simulink model "DFIG_wind_turbine_model"  (R2013a)
settings: Solver=ode45  StartTime=0.0  StopTime=10.0  RelTol=1e-3
undefined symbols (not defined in the file): c1, c2, c3, c4, c5, c6
libraries: powerlib x36
settings Model: Creator=Görkem  LastModifiedBy=Görkem

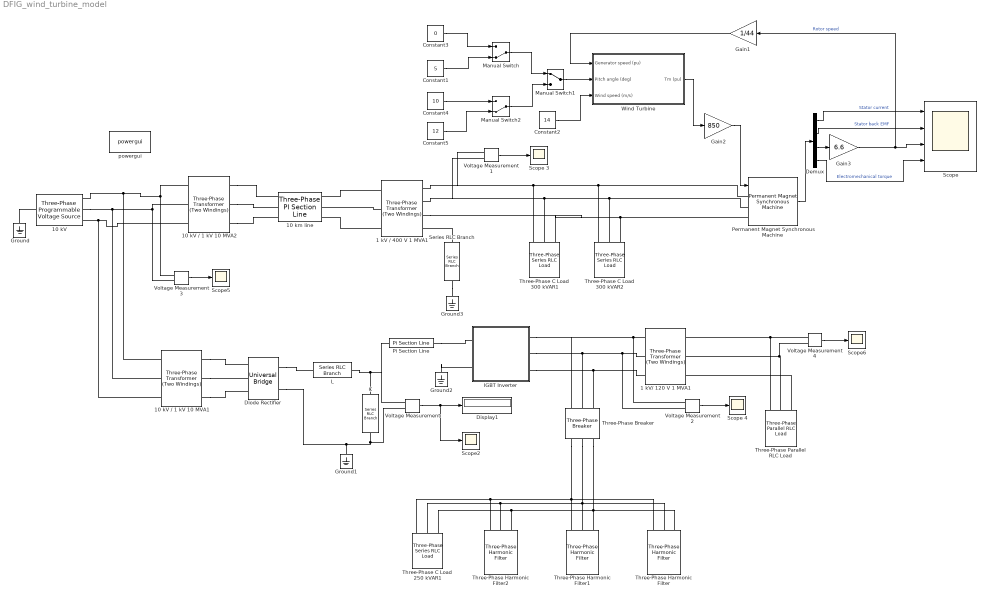
== system DFIG_wind_turbine_model ==
  1 kV / 400 V 1 MVA1 : powerlib/Elements/Three-Phase Transformer (Two Windings)  Winding1Connection=Y  UNITS=SI  NominalPower=[ 1000e3, 50 ]  Winding1=[1000 0.0023104 0.00029417]  Winding2Connection=Yn  Winding2=[400 0.0017328 0.00022063]  SetSaturation=off  Rm=577.6  Lm=1.8386  Saturation=[0 0;1.2892 2.3703;537.17 3.0024]  Hysteresis=off  DataFile='hysteresis'  SetInitialFlux=off  InitialFluxes=[1.5802 -1.5802 1.3827]  Measurements=None  MoreParameters=off  BreakLoop=off  DataType=on  TransfoNumber=1
  1 kV/ 120 V 1 MVA1 : powerlib/Elements/Three-Phase Transformer (Two Windings)  Winding1Connection=Yg  UNITS=SI  NominalPower=[ 1000000, 50 ]  Winding1=[1000 0.08712 0.011092]  Winding2Connection=Y  Winding2=[120 0.0008664 0.00011031]  SetSaturation=off  Rm=21780  Lm=69.328  Saturation=[0 0;0.29691 20.584;123.71 26.073]  Hysteresis=off  DataFile='hysteresis'  SetInitialFlux=off  InitialFluxes=[13.723 -13.723 12.007]  Measurements=None  MoreParameters=off  BreakLoop=off  DataType=on  TransfoNumber=1
  10 kV : powerlib/Electrical Sources/Three-Phase Programmable Voltage Source  PositiveSequence="[10000  0 50]"  VariationEntity=None  VariationType=Table of time-amplitude pairs  VariationTypeAlt=Step  VariationStep=0.5  VariationRate=10  VariationMagnitude=0.3  VariationFrequency=2  VariationTiming=[1 2]  VariationPhaseA=off  Amplitudes=[1 0.8 1.2 1.0]  TimeValues=[0 0.1 0.15 0.2]  HarmonicGeneration=off  HarmonicA=[3 0.2 -25 0]  HarmonicB=[2 0.15 35 2]  Timing="[0.05  3]"  BusType=swing  Pref=0  Qref=0  Qmin=-inf  Qmax=inf
  10 kV / 1 kV 10 MVA1 : powerlib/Elements/Three-Phase Transformer (Two Windings)  Winding1Connection=Y  UNITS=SI  NominalPower=[ 10e6, 50 ]  Winding1=[10000 0.0023104 0.00029417]  Winding2Connection=Y  Winding2=[1000 0.0017328 0.00022063]  SetSaturation=off  Rm=577.6  Lm=1.8386  Saturation=[0 0;1.2892 2.3703;537.17 3.0024]  Hysteresis=off  DataFile='hysteresis'  SetInitialFlux=off  InitialFluxes=[1.5802 -1.5802 1.3827]  Measurements=None  MoreParameters=off  BreakLoop=off  DataType=on  TransfoNumber=1
  10 kV / 1 kV 10 MVA2 : powerlib/Elements/Three-Phase Transformer (Two Windings)  Winding1Connection=Y  UNITS=SI  NominalPower=[ 10e6, 50 ]  Winding1=[10000 0.0023104 0.00029417]  Winding2Connection=Y  Winding2=[1000 0.0017328 0.00022063]  SetSaturation=off  Rm=577.6  Lm=1.8386  Saturation=[0 0;1.2892 2.3703;537.17 3.0024]  Hysteresis=off  DataFile='hysteresis'  SetInitialFlux=off  InitialFluxes=[1.5802 -1.5802 1.3827]  Measurements=None  MoreParameters=off  BreakLoop=off  DataType=on  TransfoNumber=1
  "10 km line " : powerlib/Elements/Three-Phase PI Section Line  LConnTagsString=a|b|c  RConnTagsString=A|B|C  Frequency=50  Resistances=[ 0.01273 0.3864]  Inductances="[ 0.9337e-3  4.1264e-3]"  Capacitances=[12.74e-9 7.751e-9]  Length=100
  C : powerlib/Elements/Series RLC Branch  LConnTagsString=__new0  RConnTagsString=__new0  BranchType=C  Resistance=1  Inductance=1e-3  SetiL0=off  InitialCurrent=0  Capacitance=0.01  Setx0=off  InitialVoltage=0  Measurements=None
  Constant1 : Constant  Value=5
  Constant2 : Constant  Value=14
  Constant3 : Constant  Value=0
  Constant4 : Constant  Value=10
  Constant5 : Constant  Value=12
  Demux : Demux
  Diode Rectifier : powerlib/Power Electronics/Universal Bridge  Arms=3  SnubberResistance=1e5  SnubberCapacitance=inf  Device=Diodes  Ron=1e-3  Lon=0  ForwardVoltages="[  0  0  ]"  ForwardVoltage=0  GTOparameters=[ 10e-6 , 20e-6 ]  IGBTparameters=[ 1e-6 , 2e-6 ]  Measurements=None  Measurements_2=None  converterType=Rectifier
  Display1 : Display
  Gain1 : Gain  Gain=1/44
  Gain2 : Gain  Gain=850
  Gain3 : Gain  Gain=6.6
  Ground{,1..3} (4 alike) : powerlib/Elements/Ground  LConnTagsString=a
  IGBT Inverter : Subsystem
  L : powerlib/Elements/Series RLC Branch  LConnTagsString=__new0  RConnTagsString=__new0  BranchType=L  Resistance=1  Inductance=3.8e-3  SetiL0=off  InitialCurrent=0  Capacitance=1e-6  Setx0=off  InitialVoltage=0  Measurements=None
  Manual Switch : ManualSwitch  CurrentSetting=0
  Manual Switch1 : ManualSwitch
  Manual Switch2 : ManualSwitch  CurrentSetting=0
  Permanent Magnet Synchronous Machine : powerlib/Machines/Permanent Magnet Synchronous Machine  NbPhases=3  FluxDistribution=Sinusoidal  RotorType=Round  MechanicalLoad=Torque Tm  PresetModel=No  ShowDetailedParameters=on  Resistance=0.0918  Inductance=8.5e-3  dqInductances=[8.5e-3,8.5e-3]  La=0.000975  MachineConstant=Flux linkage established by magnets (V.s)  Flux=0.1688  VoltageCst=122.4677  TorqueCst=1.0128  Flat=120  Mechanical=[0.003945 0.0004924 4 0]  PolePairs=4  InitialConditions=[0,0, 0,0]  InitialConditions5ph=[0 0 0 0 0 0]  TsPowergui=0  TsBlock=-1  RefAngle=90 degrees behind phase A axis (modified Park)
  Pi Section Line : powerlib/Elements/Pi Section Line  LConnTagsString=__new0  RConnTagsString=__new0  Frequency=50  Resistance=0.01273  Inductance=0.9337e-3  Capacitance=12.74e-9  Length=10  PiSections=1  Measurements=None
      settings: AttributesFormatString=\n
  Scope : Scope  NumInputPorts=4
      settings: YMin=-50000~-100000~-5~-5  YMax=50000~100000~5~5
  Scope 3 : Scope
      settings: SaveName=ScopeData3
  Scope 4 : Scope
      settings: SaveName=ScopeData4
  Scope2 : Scope
      settings: SaveName=ScopeData2
  Scope5 : Scope
      settings: SaveName=ScopeData5
  Scope6 : Scope
      settings: SaveName=ScopeData6
  Series RLC Branch : powerlib/Elements/Series RLC Branch  LConnTagsString=__new0  RConnTagsString=__new0  BranchType=R  Resistance=66  Inductance=1e-3  SetiL0=off  InitialCurrent=0  Capacitance=1e-6  Setx0=off  InitialVoltage=0  Measurements=None
  Three-Phase C Load 250 kVAR1 : powerlib/Elements/Three-Phase Series RLC Load  LConnTagsString=A|B|C  Configuration=Y (grounded)  NominalVoltage=1000  NominalFrequency=50  ActivePower=0  InductivePower=0  CapacitivePower=500000  Measurements=None  LoadType=constant Z
  Three-Phase C Load 300 kVAR1 : powerlib/Elements/Three-Phase Series RLC Load  LConnTagsString=A|B|C  Configuration=Y (floating)  NominalVoltage=380  NominalFrequency=50  ActivePower=0  InductivePower=0  CapacitivePower=300e3  Measurements=None  LoadType=constant Z
  Three-Phase C Load 300 kVAR2 : powerlib/Elements/Three-Phase Series RLC Load  LConnTagsString=A|B|C  Configuration=Y (floating)  NominalVoltage=380  NominalFrequency=50  ActivePower=0  InductivePower=0  CapacitivePower=300e3  Measurements=None  LoadType=constant Z
  Three-Phase Harmonic Filter : powerlib/Elements/Three-Phase Harmonic Filter  LConnTagsString=A|B|C  FilterType=Double-tuned  FilterConnection=Y (grounded)  ParNom=[1000 50]  Qc=500000  Fr=[5*60]  Frd=[11*50 13*50]  Q=16  Measurements=None
      settings: AttributesFormatString=\n
  Three-Phase Harmonic Filter1 : powerlib/Elements/Three-Phase Harmonic Filter  LConnTagsString=A|B|C  FilterType=C-type High-pass  FilterConnection=Y (grounded)  ParNom=[1000 50]  Qc=500000  Fr=[3*50]  Frd=[11*50 13*50]  Q=16  Measurements=None
      settings: AttributesFormatString=\n
  Three-Phase Harmonic Filter2 : powerlib/Elements/Three-Phase Harmonic Filter  LConnTagsString=A|B|C  FilterType=High-pass  FilterConnection=Y (grounded)  ParNom=[1000 50]  Qc=500000  Fr=[24*50]  Frd=[11*50 13*50]  Q=16  Measurements=None
      settings: AttributesFormatString=\n
  Three-Phase Parallel RLC Load : powerlib/Elements/Three-Phase Parallel RLC Load  LConnTagsString=A|B|C  Configuration=Y (grounded)  NominalVoltage=380  NominalFrequency=50  ActivePower=50e3  InductivePower=600  CapacitivePower=500  Measurements=None  LoadType=constant Z
  Three-Phase Breaker : powerlib/Elements/Three-Phase Breaker  InitialState=closed  SwitchA=on  SwitchB=on  SwitchC=on  SwitchTimes="[4/60  10/60]"  External=off  BreakerResistance=0.001  SnubberResistance=1e6  SnubberCapacitance=inf  Measurements=None
  Voltage Measurement{,1..4} (5 alike) : powerlib/Measurements/Voltage Measurement  PhasorSimulation=off  OutputType=Complex  PSBequivalent=0
  Wind Turbine : Subsystem  DialogController=POWERSYS.PowerSysDialog  mask(Wind Turbine){Pnom=50000, Pelec_base=56800, wind_base=14, P_wind_base=1, speed_nom=1, pitch_angle=0, DisplayTurbChar=off, c1_c6=[0.51763          116          0.4            5           21     0.006795], cp_nom=0.48, lambda_nom=8.1}
      mask prompts: Pnom "Nominal mechanical output power (W):"; Pelec_base "Base power of the electrical generator (VA):"; wind_base "Base wind speed (m/s):"; P_wind_base "Maximum power at base wind speed (pu of nominal mechanical power):"; speed_nom "Base rotational speed (p.u. of base generator speed):"; pitch_angle "Pitch angle beta to display wind-turbine power characteristics (beta >=0)  (deg):"; DisplayTurbChar "Display wind turbine power characteristics"
      mask help:
      | This block implements a variable pitch wind turbine model. The performance coefficient Cp of the turbine is the mechanical output power of the turbine divided by wind power and a function of wind speed, rotational speed, and pitch angle (beta). Cp reaches its maximum value at zero beta. Select the wind-turbine power characteristics display to plot the turbine characteristics at the specified pitch angle.
      |
      | The first input is the generator speed in per unit of the generator base speed. For a synchronous or asynchronous generator, the base speed is the synchronous speed. For a permanent-magnet generator, the base speed is defined as the speed producing nominal voltage at  no load. The second input is the blade pitch angle (beta) in degrees. The third input is the wind speed in m/s.
      |
      | The output is the torque applied to the generator shaft in per unit of the generator ratings.
      |
      | The turbine inertia must be added to the generator inertia.
      mask init:
      | %Wind turbine typical characteristic data
      | %c2=116;c3=0.4;c4=5;c5=21;
      | %Computation of c1 and c6 for lambda_nom et cpmax
      | %lambda_nom=8.1;
      | %cp_max=0.48;
      | %cp_nom=cp_max;
      | 
      | %lambda_i_nom=1/(1/lambda_nom-0.035);
      | %k_nom=-(c2*c5/lambda_i_nom-c4*c5-c2)*exp(-c5/lambda_i_nom)/lambda_nom^2;
      | %c1=cp_max/((c2/lambda_i_nom-c4)*exp(-c5/lambda_i_nom)+k_nom*lambda_nom);
      | %c6=k_nom*c1;
      | power_initmask();
      mask Help: helpview(psbhelp);
      mask Callback Pnom:
      | ParVisible={'on','on','on','on','on','on','on','off','off','off',};
      | set_param(gcb,'MaskVisibilities',ParVisible);
      | c1_c6=str2num(get_param(gcb,'c1_c6'));
      | c1=c1_c6(1);c2=c1_c6(2);c3=c1_c6(3);c4=c1_c6(4);c5=c1_c6(5);c6=c1_c6(6);
      mask Callback DisplayTurbChar:
      | DisplayTurbChar=get_param(gcb,'DisplayTurbChar');
      | 
      | if strcmp(DisplayTurbChar,'on')
      |     fig_num=figure;
      | 	clf(fig_num);
      | 	[speed_nom,wind_base,P_wind_base,pitch_angle]=getSPSmaskvalues(gcb,{'speed_nom','wind_base','P_wind_base','pitch_angle'});
      | 	[c1_c6,lambda_nom,cp_nom]=getSPSmaskvalues(gcb,{'c1_c6','lambda_nom','cp_nom'});
      | 	c1=c1_c6(1);c2=c1_c6(2);c3=c1_c6(3);c4=c1_c6(4);c5=c1_c6(5);c6=c1_c6(6);
      | 
      | 	%Wind turbine typical characteristic data
      |     %c2=116;c3=0.4;c4=5;c5=21;
      |     %Computation of c1 and c6 for lambda_nom et cpmax
      |     %lambda_nom=8.1;
      |     %cp_max=0.48;
      |     %cp_nom=cp_max;
      | 
      |     %lambda_i_nom=1/(1/lambda_nom-0.035);
      |     %k_nom=-(c2*c5/lambda_i_nom-c4*c5-c2)*exp(-c5/lambda_i_nom)/lambda_nom^2;
      |     %c1=cp_max/((c2/lambda_i_nom-c4)*exp(-c5/lambda_i_nom)+k_nom*lambda_nom);
      |     %c6=k_nom*c1;
      | 
      | 	wr_elec_pu=1e-3:0.01:1.5;;
      |     wr_mec_pu=wr_elec_pu/speed_nom;
      |     wind_max=ceil((1.2/P_wind_base)^(1/3)*wind_base);
      |     wind_min=round(((0.1)/P_wind_base)^(1/3)*wind_base);
      |     wind1=wind_min:(wind_base-wind_min)/5:wind_base;
      |     wind2=wind_base+(wind_base-wind_min)/5:(wind_base-wind_min)/5:wind_max;
      |     wind_pu=[wind1 wind2]/wind_base;
      | 
      |     for k=1:length(wind_pu)
      |         for i=1:length(wr_mec_pu);
      |             lambda_pu=wr_mec_pu(i)/wind_pu(k);
      |             lambda=lambda_pu*lambda_nom;
      |             lambda_i=1/(1/(lambda+0.08*pitch_angle)-0.035/(pitch_angle^3+1));
      |             cp=c1*(c2/lambda_i-c3*pitch_angle-c4)*exp(-c5/lambda_i)+c6*lambda;
      |             cp_pu=cp/cp_nom;
      |             Pwind_pu(k,i)=wind_pu(k)^3*cp_pu*P_wind_base;
      |         end
      |     end
      |     for k=1:length(wind_pu)
      |         plot(wr_elec_pu,Pwind_pu(k,:))
      |         hold on
      |     end
      | 
      |     plot([speed_nom,speed_nom,0],[0,P_wind_base,P_wind_base],'r--')
      |     text(speed_nom+0.01,0+0.05,sprintf('%0.4g pu',speed_nom))
      |     text(0.01,P_wind_base+0.05,sprintf('Max. power at base wind speed (%0.4g m/s) and beta = 0 deg',wind_base))
      |     for i=1:length(wind_pu),
      |         p_max(i)=max(Pwind_pu(i,:));
      |         speed(i)=wr_elec_pu(find(Pwind_pu(i,:)==p_max(i)));
      |         text(speed(i),p_max(i),sprintf('%0.4g m/s',wind_pu(i)*wind_base))
      |     end
      |     plot([0 max(wr_elec_pu)],[0 0],'--')
      | 
      |     xlabel('Turbine speed (pu of nominal generator speed)')
      |     ylabel('Turbine output power (pu of nominal mechanical power)')
      |     title(sprintf('Turbine Power Characteristics (Pitch angle beta = %0.4g deg)',pitch_angle))
      |     axis([0 max(wr_elec_pu) min(Pwind_pu(1,:)) max(P_wind_base+0.1,max(wind_pu)^3*P_wind_base+0.1)])
      |     set_param(gcb,'DisplayTurbChar','off')
      | end
      mask Display: disp('');
  powergui : powerlib/powergui  Priority=1  SimulationMode=Discrete  SolverType=Tustin  SampleTime=250e-6  frequency=60  SPID=off  DisableSnubberDevices=off  DisableRonSwitches=off  DisableVfSwitches=off  SwTol=0  Interpol=off  DisplayEquations=off  frequencyindice=50  Pbase=100e6  ErrMax=1e-4  Iterations=50  UnitsV=kV  UnitsW=MW  FunctionMessages=on  echomessages=off  HookPort=off  EnableUseOfTLC=off  x0status=blocks  RestoreLinks=warning  ResistiveCurrentMeasurement=off  Frange=[0:2:500]  Ylog=off  Xlog=on  ShowGrid=off  save=off  variable=ZData  ZoomFFT=off  StartTime=0.0  cycles=1  DisplayStyle=1  fundamental=60  FreqAxis=off  MaxFrequency=1000  frequencyindicesteady=1  RmsSteady=1  display=off  Ts=0  methode=off
  wires:
  Demux/3 -> Gain3/1
  Manual Switch1/1 -> Wind Turbine/2(Pitch angle (deg))
  Permanent Magnet Synchronous Machine/1 -> Demux/1
  Constant2/1 -> Wind Turbine/3(Wind speed (m/s))
  Wind Turbine/1(Tm (pu)) -> Gain2/1
  Gain1/1 -> Wind Turbine/1(Generator speed (pu))
  Demux/1 -> Scope/1  "Stator current"
  Demux/2 -> Scope/2  "Stator back EMF"
  Demux/4 -> Scope/4  "Electromechanical torque"
  Voltage Measurement/1 -> Display1/1, Scope2/1
  Gain2/1 -> Permanent Magnet Synchronous Machine/1
  Voltage Measurement2/1 -> Scope 4/1
  Voltage Measurement4/1 -> Scope6/1
  Voltage Measurement1/1 -> Scope 3/1
  Voltage Measurement3/1 -> Scope5/1
  Gain3/1 -> Scope/3, Gain1/1  "Rotor speed"
  Constant1/1 -> Manual Switch/2
  Constant3/1 -> Manual Switch/1
  Manual Switch/1 -> Manual Switch1/1
  Constant4/1 -> Manual Switch2/1
  Constant5/1 -> Manual Switch2/2
  Manual Switch2/1 -> Manual Switch1/2
  connections:
  L/RConn1 -- Pi Section Line/LConn1 -- Voltage Measurement/LConn1 -- C/LConn1
  Ground1/LConn1 -- Voltage Measurement/LConn2 -- C/RConn1 -- Diode Rectifier/RConn2
  Ground/LConn1 -- 10 kV/LConn1
  Pi Section Line/RConn1 -- IGBT Inverter/LConn1
  Ground2/LConn1 -- IGBT Inverter/LConn2
  Permanent Magnet Synchronous Machine/LConn2 -- Three-Phase C Load 300 kVAR2/LConn2 -- 1 kV / 400 V 1 MVA1/RConn2 -- Voltage Measurement1/LConn2 -- Three-Phase C Load 300 kVAR1/LConn2
  Three-Phase C Load 300 kVAR2/LConn3 -- Three-Phase C Load 300 kVAR1/LConn3 -- 1 kV / 400 V 1 MVA1/RConn3 -- Permanent Magnet Synchronous Machine/LConn3
  Three-Phase Parallel RLC Load/LConn2 -- Voltage Measurement4/LConn2 -- 1 kV/ 120 V 1 MVA1/RConn2
  Three-Phase Parallel RLC Load/LConn3 -- 1 kV/ 120 V 1 MVA1/RConn3
  Three-Phase Parallel RLC Load/LConn1 -- Voltage Measurement4/LConn1 -- 1 kV/ 120 V 1 MVA1/RConn1
  Voltage Measurement2/LConn1 -- IGBT Inverter/RConn1 -- Three-Phase Breaker/LConn1 -- 1 kV/ 120 V 1 MVA1/LConn1
  IGBT Inverter/RConn2 -- Three-Phase Breaker/LConn2 -- Voltage Measurement2/LConn2 -- 1 kV/ 120 V 1 MVA1/LConn2
  IGBT Inverter/RConn3 -- Three-Phase Breaker/LConn3 -- 1 kV/ 120 V 1 MVA1/LConn3
  Diode Rectifier/RConn1 -- L/LConn1
  Permanent Magnet Synchronous Machine/LConn1 -- Three-Phase C Load 300 kVAR2/LConn1 -- Voltage Measurement1/LConn1 -- 1 kV / 400 V 1 MVA1/RConn1 -- Three-Phase C Load 300 kVAR1/LConn1
  Three-Phase C Load 250 kVAR1/LConn1 -- Three-Phase Breaker/RConn1 -- Three-Phase Harmonic Filter1/LConn1 -- Three-Phase Harmonic Filter/LConn1 -- Three-Phase Harmonic Filter2/LConn1
  Three-Phase C Load 250 kVAR1/LConn2 -- Three-Phase Harmonic Filter2/LConn2 -- Three-Phase Breaker/RConn2 -- Three-Phase Harmonic Filter1/LConn2 -- Three-Phase Harmonic Filter/LConn2
  Three-Phase C Load 250 kVAR1/LConn3 -- Three-Phase Harmonic Filter2/LConn3 -- Three-Phase Breaker/RConn3 -- Three-Phase Harmonic Filter1/LConn3 -- Three-Phase Harmonic Filter/LConn3
  10 kV/RConn1 -- 10 kV / 1 kV 10 MVA1/LConn1 -- 10 kV / 1 kV 10 MVA2/LConn1 -- Voltage Measurement3/LConn1
  10 kV/RConn2 -- 10 kV / 1 kV 10 MVA1/LConn2 -- Voltage Measurement3/LConn2 -- 10 kV / 1 kV 10 MVA2/LConn2
  10 kV / 1 kV 10 MVA2/LConn3 -- 10 kV / 1 kV 10 MVA1/LConn3 -- 10 kV/RConn3
  1 kV / 400 V 1 MVA1/LConn1 -- "10 km line "/RConn1
  1 kV / 400 V 1 MVA1/LConn2 -- "10 km line "/RConn2
  1 kV / 400 V 1 MVA1/LConn3 -- "10 km line "/RConn3
  10 kV / 1 kV 10 MVA2/RConn1 -- "10 km line "/LConn1
  10 kV / 1 kV 10 MVA2/RConn2 -- "10 km line "/LConn2
  10 kV / 1 kV 10 MVA2/RConn3 -- "10 km line "/LConn3
  10 kV / 1 kV 10 MVA1/RConn1 -- Diode Rectifier/LConn1
  10 kV / 1 kV 10 MVA1/RConn2 -- Diode Rectifier/LConn2
  10 kV / 1 kV 10 MVA1/RConn3 -- Diode Rectifier/LConn3
  Series RLC Branch/LConn1 -- 1 kV / 400 V 1 MVA1/RConn4
  Series RLC Branch/RConn1 -- Ground3/LConn1

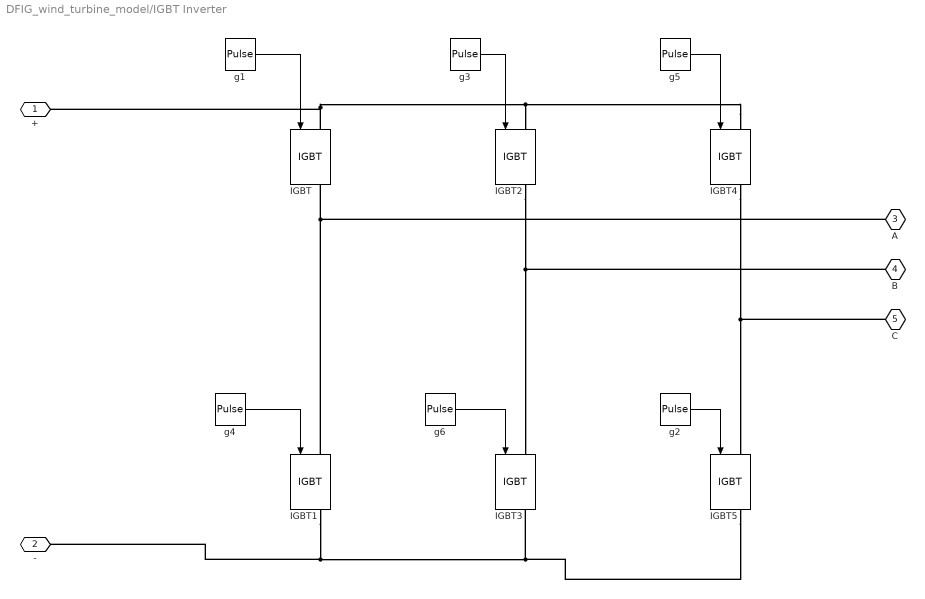
== system DFIG_wind_turbine_model/IGBT Inverter ==
  IGBT{,1..5} (6 alike) : powerlib/Power Electronics/IGBT  Ron=0.001  Lon=0  Vf=1  Tf=1e-6  Tt=2e-6  IC=0  Rs=1e5  Cs=inf  Measurements=on
  g1 : DiscretePulseGenerator  PulseType=Time based  Period=0.02  PulseWidth=50
  g2 : DiscretePulseGenerator  PulseType=Time based  Period=0.02  PulseWidth=50  PhaseDelay=0.0033
  g3 : DiscretePulseGenerator  PulseType=Time based  Period=0.02  PulseWidth=50  PhaseDelay=0.0067
  g4 : DiscretePulseGenerator  PulseType=Time based  Period=0.02  PulseWidth=50  PhaseDelay=0.01
  g5 : DiscretePulseGenerator  PulseType=Time based  Period=0.02  PulseWidth=50  PhaseDelay=0.0133
  g6 : DiscretePulseGenerator  PulseType=Time based  Period=0.02  PulseWidth=50  PhaseDelay=0.0167
  + : PMIOPort  Port=1  Side=Left
  - : PMIOPort  Port=2  Side=Left
  A : PMIOPort  Port=3  Side=Right
  B : PMIOPort  Port=4  Side=Right
  C : PMIOPort  Port=5  Side=Right
  wires:
  g4/1 -> IGBT1/1
  g2/1 -> IGBT5/1
  g6/1 -> IGBT3/1
  g1/1 -> IGBT/1
  g3/1 -> IGBT2/1
  g5/1 -> IGBT4/1
  connections:
  IGBT5/RConn1 -- IGBT3/RConn1 -- IGBT1/RConn1 -- -/RConn1
  IGBT4/LConn1 -- IGBT2/LConn1 -- IGBT/LConn1 -- +/RConn1
  IGBT2/RConn1 -- IGBT3/LConn1 -- B/RConn1
  IGBT4/RConn1 -- IGBT5/LConn1 -- C/RConn1
  IGBT1/LConn1 -- A/RConn1 -- IGBT/RConn1

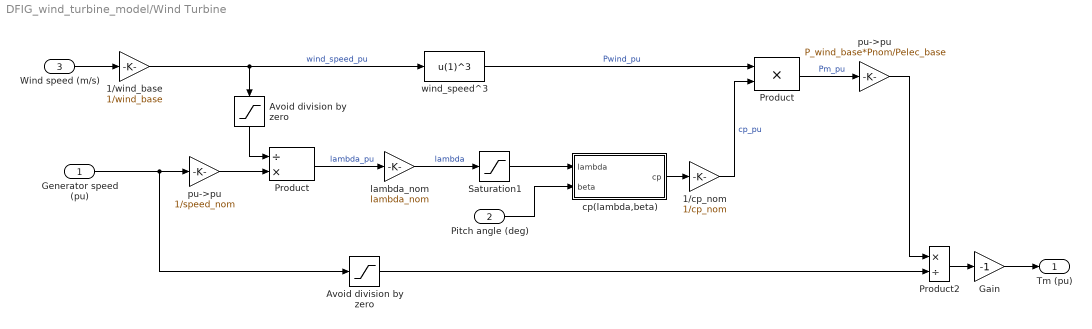
== system DFIG_wind_turbine_model/Wind Turbine ==
  Generator speed (pu) : Inport
  Pitch angle (deg) : Inport  Port=2
  Wind speed (m/s) : Inport  Port=3
  1/cp_nom : Gain  Gain=1/cp_nom  SaturateOnIntegerOverflow=on  OutDataTypeStr=Inherit: Same as input  ParamDataTypeStr=Inherit: Same as input
  1/wind_base : Gain  Gain=1/wind_base  SaturateOnIntegerOverflow=on  OutDataTypeStr=Inherit: Same as input  ParamDataTypeStr=Inherit: Same as input
  Avoid division by zero : Saturate  UpperLimit=1e6  LowerLimit=1e-6
  "Avoid division by zero " : Saturate  UpperLimit=1e6  LowerLimit=1e-6
  Gain : Gain  Gain=-1  SaturateOnIntegerOverflow=on  OutDataTypeStr=Inherit: Same as input  ParamDataTypeStr=Inherit: Same as input
  Product : Product  Inputs=/*  SaturateOnIntegerOverflow=on  OutDataTypeStr=Inherit: Same as first input
  "Product " : Product  SaturateOnIntegerOverflow=on  OutDataTypeStr=Inherit: Same as first input
  Product2 : Product  Inputs=*/  SaturateOnIntegerOverflow=on  InputSameDT=on  OutDataTypeStr=Inherit: Same as first input
  Saturation1 : Saturate  UpperLimit=inf  LowerLimit=1e-6
  cp(lambda,beta) : Subsystem
  lambda_nom : Gain  Gain=lambda_nom  SaturateOnIntegerOverflow=on  OutDataTypeStr=Inherit: Same as input  ParamDataTypeStr=Inherit: Same as input
  pu->pu : Gain  Gain=P_wind_base*Pnom/Pelec_base  SaturateOnIntegerOverflow=on  OutDataTypeStr=Inherit: Same as input  ParamDataTypeStr=Inherit: Same as input
  "pu->pu " : Gain  Gain=1/speed_nom  SaturateOnIntegerOverflow=on  OutDataTypeStr=Inherit: Same as input  ParamDataTypeStr=Inherit: Same as input
  wind_speed^3 : Fcn  Expr=u(1)^3
  Tm (pu) : Outport
  wires:
  Pitch angle (deg)/1 -> cp(lambda,beta)/2(beta)
  pu->pu/1 -> Product2/1
  cp(lambda,beta)/1(cp) -> 1/cp_nom/1
  wind_speed^3/1 -> "Product "/1  "Pwind_pu"
  Product2/1 -> Gain/1
  Avoid division by zero/1 -> Product2/2
  Wind speed (m/s)/1 -> 1/wind_base/1
  Gain/1 -> Tm (pu)/1
  Generator speed (pu)/1 -> Avoid division by zero/1, "pu->pu "/1
  "Product "/1 -> pu->pu/1  "Pm_pu"
  lambda_nom/1 -> Saturation1/1  "lambda"
  1/cp_nom/1 -> "Product "/2  "cp_pu"
  Saturation1/1 -> cp(lambda,beta)/1(lambda)
  Product/1 -> lambda_nom/1  "lambda_pu"
  1/wind_base/1 -> wind_speed^3/1, "Avoid division by zero "/1  "wind_speed_pu"
  "Avoid division by zero "/1 -> Product/1
  "pu->pu "/1 -> Product/2

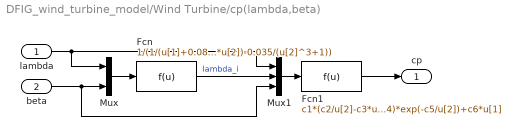
== system DFIG_wind_turbine_model/Wind Turbine/cp(lambda,beta) ==
  lambda : Inport
  beta : Inport  Port=2
  Fcn : Fcn  Expr=1/(1/(u[1]+0.08*u[2])-0.035/(u[2]^3+1))
  Fcn1 : Fcn  Expr=c1*(c2/u[2]-c3*u[3]-c4)*exp(-c5/u[2])+c6*u[1]
  Mux : Mux  Inputs=2
  Mux1 : Mux  Inputs=3
  cp : Outport
  wires:
  Fcn/1 -> Mux1/2  "lambda_i"
  Fcn1/1 -> cp/1
  lambda/1 -> Mux1/1, Mux/1
  Mux1/1 -> Fcn1/1
  beta/1 -> Mux1/3, Mux/2
  Mux/1 -> Fcn/1
